simulink model "typeA_export"  (R2017b)
settings: Solver=VariableStepAuto  StartTime=0.0  StopTime=10.0  RelTol=1e-3
values from neighbouring files (symbols this model uses):
  sys1 = sys1_exp    [check_exportvsmake.m]    (also in sumcon2mdlconst_typeA.m = sus.ss)
settings Model: Creator=ayaka  LastModifiedBy=ayaka

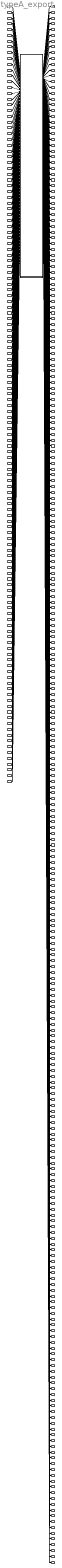
== system typeA_export ==
  axg : Inport
  ayg : Inport  Port=2
  azg : Inport  Port=3
  apitchg : Inport  Port=4
  ayawg : Inport  Port=5
  arollg : Inport  Port=6
  axHLgnd : Inport  Port=7
  ayHLgnd : Inport  Port=8
  azHLgnd : Inport  Port=9
  apitchHLgnd : Inport  Port=10
  ayawHLgnd : Inport  Port=11
  arollHLgnd : Inport  Port=12
  axHLgnd2 : Inport  Port=13
  ayHLgnd2 : Inport  Port=14
  azHLgnd2 : Inport  Port=15
  apitchHLgnd2 : Inport  Port=16
  ayawHLgnd2 : Inport  Port=17
  arollHLgnd2 : Inport  Port=18
  FxF0 : Inport  Port=19
  FzF0 : Inport  Port=20
  FyawF0 : Inport  Port=21
  FxMD : Inport  Port=22
  FyMD : Inport  Port=23
  FzMD : Inport  Port=24
  FpitchMD : Inport  Port=25
  FyawMD : Inport  Port=26
  FrollMD : Inport  Port=27
  FxF1 : Inport  Port=28
  FyF1 : Inport  Port=29
  FzF1 : Inport  Port=30
  FpitchF1 : Inport  Port=31
  FyawF1 : Inport  Port=32
  FrollF1 : Inport  Port=33
  FxF2 : Inport  Port=34
  FyF2 : Inport  Port=35
  FzF2 : Inport  Port=36
  FpitchF2 : Inport  Port=37
  FyawF2 : Inport  Port=38
  FrollF2 : Inport  Port=39
  FxF3 : Inport  Port=40
  FyF3 : Inport  Port=41
  FzF3 : Inport  Port=42
  FpitchF3 : Inport  Port=43
  FyawF3 : Inport  Port=44
  FrollF3 : Inport  Port=45
  FxBF : Inport  Port=46
  FyBF : Inport  Port=47
  FzBF : Inport  Port=48
  FpitchBF : Inport  Port=49
  FyawBF : Inport  Port=50
  FrollBF : Inport  Port=51
  FxPF : Inport  Port=52
  FyPF : Inport  Port=53
  FzPF : Inport  Port=54
  FpitchPF : Inport  Port=55
  FyawPF : Inport  Port=56
  FrollPF : Inport  Port=57
  FxMNR : Inport  Port=58
  FyMNR : Inport  Port=59
  FzMNR : Inport  Port=60
  FpitchMNR : Inport  Port=61
  FyawMNR : Inport  Port=62
  FrollMNR : Inport  Port=63
  FxMN : Inport  Port=64
  FyMN : Inport  Port=65
  FzMN : Inport  Port=66
  FpitchMN : Inport  Port=67
  FyawMN : Inport  Port=68
  FrollMN : Inport  Port=69
  FxIRM : Inport  Port=70
  FyIRM : Inport  Port=71
  FzIRM : Inport  Port=72
  FpitchIRM : Inport  Port=73
  FyawIRM : Inport  Port=74
  FrollIRM : Inport  Port=75
  FxIM : Inport  Port=76
  FyIM : Inport  Port=77
  FzIM : Inport  Port=78
  FpitchIM : Inport  Port=79
  FyawIM : Inport  Port=80
  FrollIM : Inport  Port=81
  FxRM : Inport  Port=82
  FyRM : Inport  Port=83
  FzRM : Inport  Port=84
  FpitchRM : Inport  Port=85
  FyawRM : Inport  Port=86
  FrollRM : Inport  Port=87
  FxTM : Inport  Port=88
  FyTM : Inport  Port=89
  FzTM : Inport  Port=90
  FpitchTM : Inport  Port=91
  FyawTM : Inport  Port=92
  FrollTM : Inport  Port=93
  FxHL1 : Inport  Port=94
  FyHL1 : Inport  Port=95
  FzHL1 : Inport  Port=96
  FpitchHL1 : Inport  Port=97
  FyawHL1 : Inport  Port=98
  FrollHL1 : Inport  Port=99
  FxHL2 : Inport  Port=100
  FyHL2 : Inport  Port=101
  FzHL2 : Inport  Port=102
  FpitchHL2 : Inport  Port=103
  FyawHL2 : Inport  Port=104
  FrollHL2 : Inport  Port=105
  FxHL3 : Inport  Port=106
  FyHL3 : Inport  Port=107
  FzHL3 : Inport  Port=108
  FpitchHL3 : Inport  Port=109
  FyawHL3 : Inport  Port=110
  FrollHL3 : Inport  Port=111
  FxHL21 : Inport  Port=112
  FyHL21 : Inport  Port=113
  FzHL21 : Inport  Port=114
  FpitchHL21 : Inport  Port=115
  FyawHL21 : Inport  Port=116
  FrollHL21 : Inport  Port=117
  FxHL22 : Inport  Port=118
  FyHL22 : Inport  Port=119
  FzHL22 : Inport  Port=120
  FpitchHL22 : Inport  Port=121
  FyawHL22 : Inport  Port=122
  FrollHL22 : Inport  Port=123
  FxHL23 : Inport  Port=124
  FyHL23 : Inport  Port=125
  FzHL23 : Inport  Port=126
  FpitchHL23 : Inport  Port=127
  FyawHL23 : Inport  Port=128
  FrollHL23 : Inport  Port=129
  FxJB : Inport  Port=130
  FyJB : Inport  Port=131
  FzJB : Inport  Port=132
  FpitchJB : Inport  Port=133
  FyawJB : Inport  Port=134
  FrollJB : Inport  Port=135
  Suspension : Subsystem
  xg : Outport
  yg : Outport  Port=2
  zg : Outport  Port=3
  pitchg : Outport  Port=4
  yawg : Outport  Port=5
  rollg : Outport  Port=6
  xHLgnd : Outport  Port=7
  yHLgnd : Outport  Port=8
  zHLgnd : Outport  Port=9
  pitchHLgnd : Outport  Port=10
  yawHLgnd : Outport  Port=11
  rollHLgnd : Outport  Port=12
  xHLgnd2 : Outport  Port=13
  yHLgnd2 : Outport  Port=14
  zHLgnd2 : Outport  Port=15
  pitchHLgnd2 : Outport  Port=16
  yawHLgnd2 : Outport  Port=17
  rollHLgnd2 : Outport  Port=18
  vxg : Outport  Port=19
  vyg : Outport  Port=20
  vzg : Outport  Port=21
  vpitchg : Outport  Port=22
  vyawg : Outport  Port=23
  vrollg : Outport  Port=24
  vxHLgnd : Outport  Port=25
  vyHLgnd : Outport  Port=26
  vzHLgnd : Outport  Port=27
  vpitchHLgnd : Outport  Port=28
  vyawHLgnd : Outport  Port=29
  vrollHLgnd : Outport  Port=30
  vxHLgnd2 : Outport  Port=31
  vyHLgnd2 : Outport  Port=32
  vzHLgnd2 : Outport  Port=33
  vpitchHLgnd2 : Outport  Port=34
  vyawHLgnd2 : Outport  Port=35
  vrollHLgnd2 : Outport  Port=36
  xF0 : Outport  Port=37
  zF0 : Outport  Port=38
  yawF0 : Outport  Port=39
  xMD : Outport  Port=40
  yMD : Outport  Port=41
  zMD : Outport  Port=42
  pitchMD : Outport  Port=43
  yawMD : Outport  Port=44
  rollMD : Outport  Port=45
  xF1 : Outport  Port=46
  yF1 : Outport  Port=47
  zF1 : Outport  Port=48
  pitchF1 : Outport  Port=49
  yawF1 : Outport  Port=50
  rollF1 : Outport  Port=51
  xF2 : Outport  Port=52
  yF2 : Outport  Port=53
  zF2 : Outport  Port=54
  pitchF2 : Outport  Port=55
  yawF2 : Outport  Port=56
  rollF2 : Outport  Port=57
  xF3 : Outport  Port=58
  yF3 : Outport  Port=59
  zF3 : Outport  Port=60
  pitchF3 : Outport  Port=61
  yawF3 : Outport  Port=62
  rollF3 : Outport  Port=63
  xBF : Outport  Port=64
  yBF : Outport  Port=65
  zBF : Outport  Port=66
  pitchBF : Outport  Port=67
  yawBF : Outport  Port=68
  rollBF : Outport  Port=69
  xPF : Outport  Port=70
  yPF : Outport  Port=71
  zPF : Outport  Port=72
  pitchPF : Outport  Port=73
  yawPF : Outport  Port=74
  rollPF : Outport  Port=75
  xMNR : Outport  Port=76
  yMNR : Outport  Port=77
  zMNR : Outport  Port=78
  pitchMNR : Outport  Port=79
  yawMNR : Outport  Port=80
  rollMNR : Outport  Port=81
  xMN : Outport  Port=82
  yMN : Outport  Port=83
  zMN : Outport  Port=84
  pitchMN : Outport  Port=85
  yawMN : Outport  Port=86
  rollMN : Outport  Port=87
  xIRM : Outport  Port=88
  yIRM : Outport  Port=89
  zIRM : Outport  Port=90
  pitchIRM : Outport  Port=91
  yawIRM : Outport  Port=92
  rollIRM : Outport  Port=93
  xIM : Outport  Port=94
  yIM : Outport  Port=95
  zIM : Outport  Port=96
  pitchIM : Outport  Port=97
  yawIM : Outport  Port=98
  rollIM : Outport  Port=99
  xRM : Outport  Port=100
  yRM : Outport  Port=101
  zRM : Outport  Port=102
  pitchRM : Outport  Port=103
  yawRM : Outport  Port=104
  rollRM : Outport  Port=105
  xTM : Outport  Port=106
  yTM : Outport  Port=107
  zTM : Outport  Port=108
  pitchTM : Outport  Port=109
  yawTM : Outport  Port=110
  rollTM : Outport  Port=111
  xHL1 : Outport  Port=112
  yHL1 : Outport  Port=113
  zHL1 : Outport  Port=114
  pitchHL1 : Outport  Port=115
  yawHL1 : Outport  Port=116
  rollHL1 : Outport  Port=117
  xHL2 : Outport  Port=118
  yHL2 : Outport  Port=119
  zHL2 : Outport  Port=120
  pitchHL2 : Outport  Port=121
  yawHL2 : Outport  Port=122
  rollHL2 : Outport  Port=123
  xHL3 : Outport  Port=124
  yHL3 : Outport  Port=125
  zHL3 : Outport  Port=126
  pitchHL3 : Outport  Port=127
  yawHL3 : Outport  Port=128
  rollHL3 : Outport  Port=129
  xHL21 : Outport  Port=130
  yHL21 : Outport  Port=131
  zHL21 : Outport  Port=132
  pitchHL21 : Outport  Port=133
  yawHL21 : Outport  Port=134
  rollHL21 : Outport  Port=135
  xHL22 : Outport  Port=136
  yHL22 : Outport  Port=137
  zHL22 : Outport  Port=138
  pitchHL22 : Outport  Port=139
  yawHL22 : Outport  Port=140
  rollHL22 : Outport  Port=141
  xHL23 : Outport  Port=142
  yHL23 : Outport  Port=143
  zHL23 : Outport  Port=144
  pitchHL23 : Outport  Port=145
  yawHL23 : Outport  Port=146
  rollHL23 : Outport  Port=147
  xJB : Outport  Port=148
  yJB : Outport  Port=149
  zJB : Outport  Port=150
  pitchJB : Outport  Port=151
  yawJB : Outport  Port=152
  rollJB : Outport  Port=153
  vxF0 : Outport  Port=154
  vzF0 : Outport  Port=155
  vyawF0 : Outport  Port=156
  vxMD : Outport  Port=157
  vyMD : Outport  Port=158
  vzMD : Outport  Port=159
  vpitchMD : Outport  Port=160
  vyawMD : Outport  Port=161
  vrollMD : Outport  Port=162
  vxF1 : Outport  Port=163
  vyF1 : Outport  Port=164
  vzF1 : Outport  Port=165
  vpitchF1 : Outport  Port=166
  vyawF1 : Outport  Port=167
  vrollF1 : Outport  Port=168
  vxF2 : Outport  Port=169
  vyF2 : Outport  Port=170
  vzF2 : Outport  Port=171
  vpitchF2 : Outport  Port=172
  vyawF2 : Outport  Port=173
  vrollF2 : Outport  Port=174
  vxF3 : Outport  Port=175
  vyF3 : Outport  Port=176
  vzF3 : Outport  Port=177
  vpitchF3 : Outport  Port=178
  vyawF3 : Outport  Port=179
  vrollF3 : Outport  Port=180
  vxBF : Outport  Port=181
  vyBF : Outport  Port=182
  vzBF : Outport  Port=183
  vpitchBF : Outport  Port=184
  vyawBF : Outport  Port=185
  vrollBF : Outport  Port=186
  vxPF : Outport  Port=187
  vyPF : Outport  Port=188
  vzPF : Outport  Port=189
  vpitchPF : Outport  Port=190
  vyawPF : Outport  Port=191
  vrollPF : Outport  Port=192
  vxMNR : Outport  Port=193
  vyMNR : Outport  Port=194
  vzMNR : Outport  Port=195
  vpitchMNR : Outport  Port=196
  vyawMNR : Outport  Port=197
  vrollMNR : Outport  Port=198
  vxMN : Outport  Port=199
  vyMN : Outport  Port=200
  vzMN : Outport  Port=201
  vpitchMN : Outport  Port=202
  vyawMN : Outport  Port=203
  vrollMN : Outport  Port=204
  vxIRM : Outport  Port=205
  vyIRM : Outport  Port=206
  vzIRM : Outport  Port=207
  vpitchIRM : Outport  Port=208
  vyawIRM : Outport  Port=209
  vrollIRM : Outport  Port=210
  vxIM : Outport  Port=211
  vyIM : Outport  Port=212
  vzIM : Outport  Port=213
  vpitchIM : Outport  Port=214
  vyawIM : Outport  Port=215
  vrollIM : Outport  Port=216
  vxRM : Outport  Port=217
  vyRM : Outport  Port=218
  vzRM : Outport  Port=219
  vpitchRM : Outport  Port=220
  vyawRM : Outport  Port=221
  vrollRM : Outport  Port=222
  vxTM : Outport  Port=223
  vyTM : Outport  Port=224
  vzTM : Outport  Port=225
  vpitchTM : Outport  Port=226
  vyawTM : Outport  Port=227
  vrollTM : Outport  Port=228
  vxHL1 : Outport  Port=229
  vyHL1 : Outport  Port=230
  vzHL1 : Outport  Port=231
  vpitchHL1 : Outport  Port=232
  vyawHL1 : Outport  Port=233
  vrollHL1 : Outport  Port=234
  vxHL2 : Outport  Port=235
  vyHL2 : Outport  Port=236
  vzHL2 : Outport  Port=237
  vpitchHL2 : Outport  Port=238
  vyawHL2 : Outport  Port=239
  vrollHL2 : Outport  Port=240
  vxHL3 : Outport  Port=241
  vyHL3 : Outport  Port=242
  vzHL3 : Outport  Port=243
  vpitchHL3 : Outport  Port=244
  vyawHL3 : Outport  Port=245
  vrollHL3 : Outport  Port=246
  vxHL21 : Outport  Port=247
  vyHL21 : Outport  Port=248
  vzHL21 : Outport  Port=249
  vpitchHL21 : Outport  Port=250
  vyawHL21 : Outport  Port=251
  vrollHL21 : Outport  Port=252
  vxHL22 : Outport  Port=253
  vyHL22 : Outport  Port=254
  vzHL22 : Outport  Port=255
  vpitchHL22 : Outport  Port=256
  vyawHL22 : Outport  Port=257
  vrollHL22 : Outport  Port=258
  vxHL23 : Outport  Port=259
  vyHL23 : Outport  Port=260
  vzHL23 : Outport  Port=261
  vpitchHL23 : Outport  Port=262
  vyawHL23 : Outport  Port=263
  vrollHL23 : Outport  Port=264
  vxJB : Outport  Port=265
  vyJB : Outport  Port=266
  vzJB : Outport  Port=267
  vpitchJB : Outport  Port=268
  vyawJB : Outport  Port=269
  vrollJB : Outport  Port=270
  wires:
  axg/1 -> Suspension/1(axg)
  ayg/1 -> Suspension/2(ayg)
  azg/1 -> Suspension/3(azg)
  apitchg/1 -> Suspension/4(apitchg)
  ayawg/1 -> Suspension/5(ayawg)
  arollg/1 -> Suspension/6(arollg)
  axHLgnd/1 -> Suspension/7(axHLgnd)
  ayHLgnd/1 -> Suspension/8(ayHLgnd)
  azHLgnd/1 -> Suspension/9(azHLgnd)
  apitchHLgnd/1 -> Suspension/10(apitchHLgnd)
  ayawHLgnd/1 -> Suspension/11(ayawHLgnd)
  arollHLgnd/1 -> Suspension/12(arollHLgnd)
  axHLgnd2/1 -> Suspension/13(axHLgnd2)
  ayHLgnd2/1 -> Suspension/14(ayHLgnd2)
  azHLgnd2/1 -> Suspension/15(azHLgnd2)
  apitchHLgnd2/1 -> Suspension/16(apitchHLgnd2)
  ayawHLgnd2/1 -> Suspension/17(ayawHLgnd2)
  arollHLgnd2/1 -> Suspension/18(arollHLgnd2)
  FxF0/1 -> Suspension/19(FxF0)
  FzF0/1 -> Suspension/20(FzF0)
  FyawF0/1 -> Suspension/21(FyawF0)
  FxMD/1 -> Suspension/22(FxMD)
  FyMD/1 -> Suspension/23(FyMD)
  FzMD/1 -> Suspension/24(FzMD)
  FpitchMD/1 -> Suspension/25(FpitchMD)
  FyawMD/1 -> Suspension/26(FyawMD)
  FrollMD/1 -> Suspension/27(FrollMD)
  FxF1/1 -> Suspension/28(FxF1)
  FyF1/1 -> Suspension/29(FyF1)
  FzF1/1 -> Suspension/30(FzF1)
  FpitchF1/1 -> Suspension/31(FpitchF1)
  FyawF1/1 -> Suspension/32(FyawF1)
  FrollF1/1 -> Suspension/33(FrollF1)
  FxF2/1 -> Suspension/34(FxF2)
  FyF2/1 -> Suspension/35(FyF2)
  FzF2/1 -> Suspension/36(FzF2)
  FpitchF2/1 -> Suspension/37(FpitchF2)
  FyawF2/1 -> Suspension/38(FyawF2)
  FrollF2/1 -> Suspension/39(FrollF2)
  FxF3/1 -> Suspension/40(FxF3)
  FyF3/1 -> Suspension/41(FyF3)
  FzF3/1 -> Suspension/42(FzF3)
  FpitchF3/1 -> Suspension/43(FpitchF3)
  FyawF3/1 -> Suspension/44(FyawF3)
  FrollF3/1 -> Suspension/45(FrollF3)
  FxBF/1 -> Suspension/46(FxBF)
  FyBF/1 -> Suspension/47(FyBF)
  FzBF/1 -> Suspension/48(FzBF)
  FpitchBF/1 -> Suspension/49(FpitchBF)
  FyawBF/1 -> Suspension/50(FyawBF)
  FrollBF/1 -> Suspension/51(FrollBF)
  FxPF/1 -> Suspension/52(FxPF)
  FyPF/1 -> Suspension/53(FyPF)
  FzPF/1 -> Suspension/54(FzPF)
  FpitchPF/1 -> Suspension/55(FpitchPF)
  FyawPF/1 -> Suspension/56(FyawPF)
  FrollPF/1 -> Suspension/57(FrollPF)
  FxMNR/1 -> Suspension/58(FxMNR)
  FyMNR/1 -> Suspension/59(FyMNR)
  FzMNR/1 -> Suspension/60(FzMNR)
  FpitchMNR/1 -> Suspension/61(FpitchMNR)
  FyawMNR/1 -> Suspension/62(FyawMNR)
  FrollMNR/1 -> Suspension/63(FrollMNR)
  FxMN/1 -> Suspension/64(FxMN)
  FyMN/1 -> Suspension/65(FyMN)
  FzMN/1 -> Suspension/66(FzMN)
  FpitchMN/1 -> Suspension/67(FpitchMN)
  FyawMN/1 -> Suspension/68(FyawMN)
  FrollMN/1 -> Suspension/69(FrollMN)
  FxIRM/1 -> Suspension/70(FxIRM)
  FyIRM/1 -> Suspension/71(FyIRM)
  FzIRM/1 -> Suspension/72(FzIRM)
  FpitchIRM/1 -> Suspension/73(FpitchIRM)
  FyawIRM/1 -> Suspension/74(FyawIRM)
  FrollIRM/1 -> Suspension/75(FrollIRM)
  FxIM/1 -> Suspension/76(FxIM)
  FyIM/1 -> Suspension/77(FyIM)
  FzIM/1 -> Suspension/78(FzIM)
  FpitchIM/1 -> Suspension/79(FpitchIM)
  FyawIM/1 -> Suspension/80(FyawIM)
  FrollIM/1 -> Suspension/81(FrollIM)
  FxRM/1 -> Suspension/82(FxRM)
  FyRM/1 -> Suspension/83(FyRM)
  FzRM/1 -> Suspension/84(FzRM)
  FpitchRM/1 -> Suspension/85(FpitchRM)
  FyawRM/1 -> Suspension/86(FyawRM)
  FrollRM/1 -> Suspension/87(FrollRM)
  FxTM/1 -> Suspension/88(FxTM)
  FyTM/1 -> Suspension/89(FyTM)
  FzTM/1 -> Suspension/90(FzTM)
  FpitchTM/1 -> Suspension/91(FpitchTM)
  FyawTM/1 -> Suspension/92(FyawTM)
  FrollTM/1 -> Suspension/93(FrollTM)
  FxHL1/1 -> Suspension/94(FxHL1)
  FyHL1/1 -> Suspension/95(FyHL1)
  FzHL1/1 -> Suspension/96(FzHL1)
  FpitchHL1/1 -> Suspension/97(FpitchHL1)
  FyawHL1/1 -> Suspension/98(FyawHL1)
  FrollHL1/1 -> Suspension/99(FrollHL1)
  FxHL2/1 -> Suspension/100(FxHL2)
  FyHL2/1 -> Suspension/101(FyHL2)
  FzHL2/1 -> Suspension/102(FzHL2)
  FpitchHL2/1 -> Suspension/103(FpitchHL2)
  FyawHL2/1 -> Suspension/104(FyawHL2)
  FrollHL2/1 -> Suspension/105(FrollHL2)
  FxHL3/1 -> Suspension/106(FxHL3)
  FyHL3/1 -> Suspension/107(FyHL3)
  FzHL3/1 -> Suspension/108(FzHL3)
  FpitchHL3/1 -> Suspension/109(FpitchHL3)
  FyawHL3/1 -> Suspension/110(FyawHL3)
  FrollHL3/1 -> Suspension/111(FrollHL3)
  FxHL21/1 -> Suspension/112(FxHL21)
  FyHL21/1 -> Suspension/113(FyHL21)
  FzHL21/1 -> Suspension/114(FzHL21)
  FpitchHL21/1 -> Suspension/115(FpitchHL21)
  FyawHL21/1 -> Suspension/116(FyawHL21)
  FrollHL21/1 -> Suspension/117(FrollHL21)
  FxHL22/1 -> Suspension/118(FxHL22)
  FyHL22/1 -> Suspension/119(FyHL22)
  FzHL22/1 -> Suspension/120(FzHL22)
  FpitchHL22/1 -> Suspension/121(FpitchHL22)
  FyawHL22/1 -> Suspension/122(FyawHL22)
  FrollHL22/1 -> Suspension/123(FrollHL22)
  FxHL23/1 -> Suspension/124(FxHL23)
  FyHL23/1 -> Suspension/125(FyHL23)
  FzHL23/1 -> Suspension/126(FzHL23)
  FpitchHL23/1 -> Suspension/127(FpitchHL23)
  FyawHL23/1 -> Suspension/128(FyawHL23)
  FrollHL23/1 -> Suspension/129(FrollHL23)
  FxJB/1 -> Suspension/130(FxJB)
  FyJB/1 -> Suspension/131(FyJB)
  FzJB/1 -> Suspension/132(FzJB)
  FpitchJB/1 -> Suspension/133(FpitchJB)
  FyawJB/1 -> Suspension/134(FyawJB)
  FrollJB/1 -> Suspension/135(FrollJB)
  Suspension/1(xg) -> xg/1
  Suspension/2(yg) -> yg/1
  Suspension/3(zg) -> zg/1
  Suspension/4(pitchg) -> pitchg/1
  Suspension/5(yawg) -> yawg/1
  Suspension/6(rollg) -> rollg/1
  Suspension/7(xHLgnd) -> xHLgnd/1
  Suspension/8(yHLgnd) -> yHLgnd/1
  Suspension/9(zHLgnd) -> zHLgnd/1
  Suspension/10(pitchHLgnd) -> pitchHLgnd/1
  Suspension/11(yawHLgnd) -> yawHLgnd/1
  Suspension/12(rollHLgnd) -> rollHLgnd/1
  Suspension/13(xHLgnd2) -> xHLgnd2/1
  Suspension/14(yHLgnd2) -> yHLgnd2/1
  Suspension/15(zHLgnd2) -> zHLgnd2/1
  Suspension/16(pitchHLgnd2) -> pitchHLgnd2/1
  Suspension/17(yawHLgnd2) -> yawHLgnd2/1
  Suspension/18(rollHLgnd2) -> rollHLgnd2/1
  Suspension/19(vxg) -> vxg/1
  Suspension/20(vyg) -> vyg/1
  Suspension/21(vzg) -> vzg/1
  Suspension/22(vpitchg) -> vpitchg/1
  Suspension/23(vyawg) -> vyawg/1
  Suspension/24(vrollg) -> vrollg/1
  Suspension/25(vxHLgnd) -> vxHLgnd/1
  Suspension/26(vyHLgnd) -> vyHLgnd/1
  Suspension/27(vzHLgnd) -> vzHLgnd/1
  Suspension/28(vpitchHLgnd) -> vpitchHLgnd/1
  Suspension/29(vyawHLgnd) -> vyawHLgnd/1
  Suspension/30(vrollHLgnd) -> vrollHLgnd/1
  Suspension/31(vxHLgnd2) -> vxHLgnd2/1
  Suspension/32(vyHLgnd2) -> vyHLgnd2/1
  Suspension/33(vzHLgnd2) -> vzHLgnd2/1
  Suspension/34(vpitchHLgnd2) -> vpitchHLgnd2/1
  Suspension/35(vyawHLgnd2) -> vyawHLgnd2/1
  Suspension/36(vrollHLgnd2) -> vrollHLgnd2/1
  Suspension/37(xF0) -> xF0/1
  Suspension/38(zF0) -> zF0/1
  Suspension/39(yawF0) -> yawF0/1
  Suspension/40(xMD) -> xMD/1
  Suspension/41(yMD) -> yMD/1
  Suspension/42(zMD) -> zMD/1
  Suspension/43(pitchMD) -> pitchMD/1
  Suspension/44(yawMD) -> yawMD/1
  Suspension/45(rollMD) -> rollMD/1
  Suspension/46(xF1) -> xF1/1
  Suspension/47(yF1) -> yF1/1
  Suspension/48(zF1) -> zF1/1
  Suspension/49(pitchF1) -> pitchF1/1
  Suspension/50(yawF1) -> yawF1/1
  Suspension/51(rollF1) -> rollF1/1
  Suspension/52(xF2) -> xF2/1
  Suspension/53(yF2) -> yF2/1
  Suspension/54(zF2) -> zF2/1
  Suspension/55(pitchF2) -> pitchF2/1
  Suspension/56(yawF2) -> yawF2/1
  Suspension/57(rollF2) -> rollF2/1
  Suspension/58(xF3) -> xF3/1
  Suspension/59(yF3) -> yF3/1
  Suspension/60(zF3) -> zF3/1
  Suspension/61(pitchF3) -> pitchF3/1
  Suspension/62(yawF3) -> yawF3/1
  Suspension/63(rollF3) -> rollF3/1
  Suspension/64(xBF) -> xBF/1
  Suspension/65(yBF) -> yBF/1
  Suspension/66(zBF) -> zBF/1
  Suspension/67(pitchBF) -> pitchBF/1
  Suspension/68(yawBF) -> yawBF/1
  Suspension/69(rollBF) -> rollBF/1
  Suspension/70(xPF) -> xPF/1
  Suspension/71(yPF) -> yPF/1
  Suspension/72(zPF) -> zPF/1
  Suspension/73(pitchPF) -> pitchPF/1
  Suspension/74(yawPF) -> yawPF/1
  Suspension/75(rollPF) -> rollPF/1
  Suspension/76(xMNR) -> xMNR/1
  Suspension/77(yMNR) -> yMNR/1
  Suspension/78(zMNR) -> zMNR/1
  Suspension/79(pitchMNR) -> pitchMNR/1
  Suspension/80(yawMNR) -> yawMNR/1
  Suspension/81(rollMNR) -> rollMNR/1
  Suspension/82(xMN) -> xMN/1
  Suspension/83(yMN) -> yMN/1
  Suspension/84(zMN) -> zMN/1
  Suspension/85(pitchMN) -> pitchMN/1
  Suspension/86(yawMN) -> yawMN/1
  Suspension/87(rollMN) -> rollMN/1
  Suspension/88(xIRM) -> xIRM/1
  Suspension/89(yIRM) -> yIRM/1
  Suspension/90(zIRM) -> zIRM/1
  Suspension/91(pitchIRM) -> pitchIRM/1
  Suspension/92(yawIRM) -> yawIRM/1
  Suspension/93(rollIRM) -> rollIRM/1
  Suspension/94(xIM) -> xIM/1
  Suspension/95(yIM) -> yIM/1
  Suspension/96(zIM) -> zIM/1
  Suspension/97(pitchIM) -> pitchIM/1
  Suspension/98(yawIM) -> yawIM/1
  Suspension/99(rollIM) -> rollIM/1
  Suspension/100(xRM) -> xRM/1
  Suspension/101(yRM) -> yRM/1
  Suspension/102(zRM) -> zRM/1
  Suspension/103(pitchRM) -> pitchRM/1
  Suspension/104(yawRM) -> yawRM/1
  Suspension/105(rollRM) -> rollRM/1
  Suspension/106(xTM) -> xTM/1
  Suspension/107(yTM) -> yTM/1
  Suspension/108(zTM) -> zTM/1
  Suspension/109(pitchTM) -> pitchTM/1
  Suspension/110(yawTM) -> yawTM/1
  Suspension/111(rollTM) -> rollTM/1
  Suspension/112(xHL1) -> xHL1/1
  Suspension/113(yHL1) -> yHL1/1
  Suspension/114(zHL1) -> zHL1/1
  Suspension/115(pitchHL1) -> pitchHL1/1
  Suspension/116(yawHL1) -> yawHL1/1
  Suspension/117(rollHL1) -> rollHL1/1
  Suspension/118(xHL2) -> xHL2/1
  Suspension/119(yHL2) -> yHL2/1
  Suspension/120(zHL2) -> zHL2/1
  Suspension/121(pitchHL2) -> pitchHL2/1
  Suspension/122(yawHL2) -> yawHL2/1
  Suspension/123(rollHL2) -> rollHL2/1
  Suspension/124(xHL3) -> xHL3/1
  Suspension/125(yHL3) -> yHL3/1
  Suspension/126(zHL3) -> zHL3/1
  Suspension/127(pitchHL3) -> pitchHL3/1
  Suspension/128(yawHL3) -> yawHL3/1
  Suspension/129(rollHL3) -> rollHL3/1
  Suspension/130(xHL21) -> xHL21/1
  Suspension/131(yHL21) -> yHL21/1
  Suspension/132(zHL21) -> zHL21/1
  Suspension/133(pitchHL21) -> pitchHL21/1
  Suspension/134(yawHL21) -> yawHL21/1
  Suspension/135(rollHL21) -> rollHL21/1
  Suspension/136(xHL22) -> xHL22/1
  Suspension/137(yHL22) -> yHL22/1
  Suspension/138(zHL22) -> zHL22/1
  Suspension/139(pitchHL22) -> pitchHL22/1
  Suspension/140(yawHL22) -> yawHL22/1
  Suspension/141(rollHL22) -> rollHL22/1
  Suspension/142(xHL23) -> xHL23/1
  Suspension/143(yHL23) -> yHL23/1
  Suspension/144(zHL23) -> zHL23/1
  Suspension/145(pitchHL23) -> pitchHL23/1
  Suspension/146(yawHL23) -> yawHL23/1
  Suspension/147(rollHL23) -> rollHL23/1
  Suspension/148(xJB) -> xJB/1
  Suspension/149(yJB) -> yJB/1
  Suspension/150(zJB) -> zJB/1
  Suspension/151(pitchJB) -> pitchJB/1
  Suspension/152(yawJB) -> yawJB/1
  Suspension/153(rollJB) -> rollJB/1
  Suspension/154(vxF0) -> vxF0/1
  Suspension/155(vzF0) -> vzF0/1
  Suspension/156(vyawF0) -> vyawF0/1
  Suspension/157(vxMD) -> vxMD/1
  Suspension/158(vyMD) -> vyMD/1
  Suspension/159(vzMD) -> vzMD/1
  Suspension/160(vpitchMD) -> vpitchMD/1
  Suspension/161(vyawMD) -> vyawMD/1
  Suspension/162(vrollMD) -> vrollMD/1
  Suspension/163(vxF1) -> vxF1/1
  Suspension/164(vyF1) -> vyF1/1
  Suspension/165(vzF1) -> vzF1/1
  Suspension/166(vpitchF1) -> vpitchF1/1
  Suspension/167(vyawF1) -> vyawF1/1
  Suspension/168(vrollF1) -> vrollF1/1
  Suspension/169(vxF2) -> vxF2/1
  Suspension/170(vyF2) -> vyF2/1
  Suspension/171(vzF2) -> vzF2/1
  Suspension/172(vpitchF2) -> vpitchF2/1
  Suspension/173(vyawF2) -> vyawF2/1
  Suspension/174(vrollF2) -> vrollF2/1
  Suspension/175(vxF3) -> vxF3/1
  Suspension/176(vyF3) -> vyF3/1
  Suspension/177(vzF3) -> vzF3/1
  Suspension/178(vpitchF3) -> vpitchF3/1
  Suspension/179(vyawF3) -> vyawF3/1
  Suspension/180(vrollF3) -> vrollF3/1
  Suspension/181(vxBF) -> vxBF/1
  Suspension/182(vyBF) -> vyBF/1
  Suspension/183(vzBF) -> vzBF/1
  Suspension/184(vpitchBF) -> vpitchBF/1
  Suspension/185(vyawBF) -> vyawBF/1
  Suspension/186(vrollBF) -> vrollBF/1
  Suspension/187(vxPF) -> vxPF/1
  Suspension/188(vyPF) -> vyPF/1
  Suspension/189(vzPF) -> vzPF/1
  Suspension/190(vpitchPF) -> vpitchPF/1
  Suspension/191(vyawPF) -> vyawPF/1
  Suspension/192(vrollPF) -> vrollPF/1
  Suspension/193(vxMNR) -> vxMNR/1
  Suspension/194(vyMNR) -> vyMNR/1
  Suspension/195(vzMNR) -> vzMNR/1
  Suspension/196(vpitchMNR) -> vpitchMNR/1
  Suspension/197(vyawMNR) -> vyawMNR/1
  Suspension/198(vrollMNR) -> vrollMNR/1
  Suspension/199(vxMN) -> vxMN/1
  Suspension/200(vyMN) -> vyMN/1
  Suspension/201(vzMN) -> vzMN/1
  Suspension/202(vpitchMN) -> vpitchMN/1
  Suspension/203(vyawMN) -> vyawMN/1
  Suspension/204(vrollMN) -> vrollMN/1
  Suspension/205(vxIRM) -> vxIRM/1
  Suspension/206(vyIRM) -> vyIRM/1
  Suspension/207(vzIRM) -> vzIRM/1
  Suspension/208(vpitchIRM) -> vpitchIRM/1
  Suspension/209(vyawIRM) -> vyawIRM/1
  Suspension/210(vrollIRM) -> vrollIRM/1
  Suspension/211(vxIM) -> vxIM/1
  Suspension/212(vyIM) -> vyIM/1
  Suspension/213(vzIM) -> vzIM/1
  Suspension/214(vpitchIM) -> vpitchIM/1
  Suspension/215(vyawIM) -> vyawIM/1
  Suspension/216(vrollIM) -> vrollIM/1
  Suspension/217(vxRM) -> vxRM/1
  Suspension/218(vyRM) -> vyRM/1
  Suspension/219(vzRM) -> vzRM/1
  Suspension/220(vpitchRM) -> vpitchRM/1
  Suspension/221(vyawRM) -> vyawRM/1
  Suspension/222(vrollRM) -> vrollRM/1
  Suspension/223(vxTM) -> vxTM/1
  Suspension/224(vyTM) -> vyTM/1
  Suspension/225(vzTM) -> vzTM/1
  Suspension/226(vpitchTM) -> vpitchTM/1
  Suspension/227(vyawTM) -> vyawTM/1
  Suspension/228(vrollTM) -> vrollTM/1
  Suspension/229(vxHL1) -> vxHL1/1
  Suspension/230(vyHL1) -> vyHL1/1
  Suspension/231(vzHL1) -> vzHL1/1
  Suspension/232(vpitchHL1) -> vpitchHL1/1
  Suspension/233(vyawHL1) -> vyawHL1/1
  Suspension/234(vrollHL1) -> vrollHL1/1
  Suspension/235(vxHL2) -> vxHL2/1
  Suspension/236(vyHL2) -> vyHL2/1
  Suspension/237(vzHL2) -> vzHL2/1
  Suspension/238(vpitchHL2) -> vpitchHL2/1
  Suspension/239(vyawHL2) -> vyawHL2/1
  Suspension/240(vrollHL2) -> vrollHL2/1
  Suspension/241(vxHL3) -> vxHL3/1
  Suspension/242(vyHL3) -> vyHL3/1
  Suspension/243(vzHL3) -> vzHL3/1
  Suspension/244(vpitchHL3) -> vpitchHL3/1
  Suspension/245(vyawHL3) -> vyawHL3/1
  Suspension/246(vrollHL3) -> vrollHL3/1
  Suspension/247(vxHL21) -> vxHL21/1
  Suspension/248(vyHL21) -> vyHL21/1
  Suspension/249(vzHL21) -> vzHL21/1
  Suspension/250(vpitchHL21) -> vpitchHL21/1
  Suspension/251(vyawHL21) -> vyawHL21/1
  Suspension/252(vrollHL21) -> vrollHL21/1
  Suspension/253(vxHL22) -> vxHL22/1
  Suspension/254(vyHL22) -> vyHL22/1
  Suspension/255(vzHL22) -> vzHL22/1
  Suspension/256(vpitchHL22) -> vpitchHL22/1
  Suspension/257(vyawHL22) -> vyawHL22/1
  Suspension/258(vrollHL22) -> vrollHL22/1
  Suspension/259(vxHL23) -> vxHL23/1
  Suspension/260(vyHL23) -> vyHL23/1
  Suspension/261(vzHL23) -> vzHL23/1
  Suspension/262(vpitchHL23) -> vpitchHL23/1
  Suspension/263(vyawHL23) -> vyawHL23/1
  Suspension/264(vrollHL23) -> vrollHL23/1
  Suspension/265(vxJB) -> vxJB/1
  Suspension/266(vyJB) -> vyJB/1
  Suspension/267(vzJB) -> vzJB/1
  Suspension/268(vpitchJB) -> vpitchJB/1
  Suspension/269(vyawJB) -> vyawJB/1
  Suspension/270(vrollJB) -> vrollJB/1

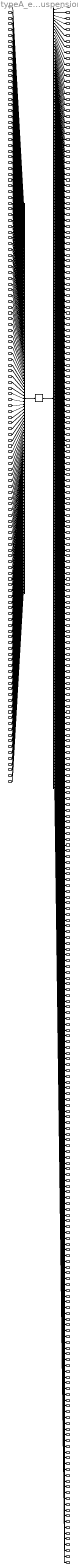
== system typeA_export/Suspension ==
  axg : Inport
  ayg : Inport  Port=2
  azg : Inport  Port=3
  apitchg : Inport  Port=4
  ayawg : Inport  Port=5
  arollg : Inport  Port=6
  axHLgnd : Inport  Port=7
  ayHLgnd : Inport  Port=8
  azHLgnd : Inport  Port=9
  apitchHLgnd : Inport  Port=10
  ayawHLgnd : Inport  Port=11
  arollHLgnd : Inport  Port=12
  axHLgnd2 : Inport  Port=13
  ayHLgnd2 : Inport  Port=14
  azHLgnd2 : Inport  Port=15
  apitchHLgnd2 : Inport  Port=16
  ayawHLgnd2 : Inport  Port=17
  arollHLgnd2 : Inport  Port=18
  FxF0 : Inport  Port=19
  FzF0 : Inport  Port=20
  FyawF0 : Inport  Port=21
  FxMD : Inport  Port=22
  FyMD : Inport  Port=23
  FzMD : Inport  Port=24
  FpitchMD : Inport  Port=25
  FyawMD : Inport  Port=26
  FrollMD : Inport  Port=27
  FxF1 : Inport  Port=28
  FyF1 : Inport  Port=29
  FzF1 : Inport  Port=30
  FpitchF1 : Inport  Port=31
  FyawF1 : Inport  Port=32
  FrollF1 : Inport  Port=33
  FxF2 : Inport  Port=34
  FyF2 : Inport  Port=35
  FzF2 : Inport  Port=36
  FpitchF2 : Inport  Port=37
  FyawF2 : Inport  Port=38
  FrollF2 : Inport  Port=39
  FxF3 : Inport  Port=40
  FyF3 : Inport  Port=41
  FzF3 : Inport  Port=42
  FpitchF3 : Inport  Port=43
  FyawF3 : Inport  Port=44
  FrollF3 : Inport  Port=45
  FxBF : Inport  Port=46
  FyBF : Inport  Port=47
  FzBF : Inport  Port=48
  FpitchBF : Inport  Port=49
  FyawBF : Inport  Port=50
  FrollBF : Inport  Port=51
  FxPF : Inport  Port=52
  FyPF : Inport  Port=53
  FzPF : Inport  Port=54
  FpitchPF : Inport  Port=55
  FyawPF : Inport  Port=56
  FrollPF : Inport  Port=57
  FxMNR : Inport  Port=58
  FyMNR : Inport  Port=59
  FzMNR : Inport  Port=60
  FpitchMNR : Inport  Port=61
  FyawMNR : Inport  Port=62
  FrollMNR : Inport  Port=63
  FxMN : Inport  Port=64
  FyMN : Inport  Port=65
  FzMN : Inport  Port=66
  FpitchMN : Inport  Port=67
  FyawMN : Inport  Port=68
  FrollMN : Inport  Port=69
  FxIRM : Inport  Port=70
  FyIRM : Inport  Port=71
  FzIRM : Inport  Port=72
  FpitchIRM : Inport  Port=73
  FyawIRM : Inport  Port=74
  FrollIRM : Inport  Port=75
  FxIM : Inport  Port=76
  FyIM : Inport  Port=77
  FzIM : Inport  Port=78
  FpitchIM : Inport  Port=79
  FyawIM : Inport  Port=80
  FrollIM : Inport  Port=81
  FxRM : Inport  Port=82
  FyRM : Inport  Port=83
  FzRM : Inport  Port=84
  FpitchRM : Inport  Port=85
  FyawRM : Inport  Port=86
  FrollRM : Inport  Port=87
  FxTM : Inport  Port=88
  FyTM : Inport  Port=89
  FzTM : Inport  Port=90
  FpitchTM : Inport  Port=91
  FyawTM : Inport  Port=92
  FrollTM : Inport  Port=93
  FxHL1 : Inport  Port=94
  FyHL1 : Inport  Port=95
  FzHL1 : Inport  Port=96
  FpitchHL1 : Inport  Port=97
  FyawHL1 : Inport  Port=98
  FrollHL1 : Inport  Port=99
  FxHL2 : Inport  Port=100
  FyHL2 : Inport  Port=101
  FzHL2 : Inport  Port=102
  FpitchHL2 : Inport  Port=103
  FyawHL2 : Inport  Port=104
  FrollHL2 : Inport  Port=105
  FxHL3 : Inport  Port=106
  FyHL3 : Inport  Port=107
  FzHL3 : Inport  Port=108
  FpitchHL3 : Inport  Port=109
  FyawHL3 : Inport  Port=110
  FrollHL3 : Inport  Port=111
  FxHL21 : Inport  Port=112
  FyHL21 : Inport  Port=113
  FzHL21 : Inport  Port=114
  FpitchHL21 : Inport  Port=115
  FyawHL21 : Inport  Port=116
  FrollHL21 : Inport  Port=117
  FxHL22 : Inport  Port=118
  FyHL22 : Inport  Port=119
  FzHL22 : Inport  Port=120
  FpitchHL22 : Inport  Port=121
  FyawHL22 : Inport  Port=122
  FrollHL22 : Inport  Port=123
  FxHL23 : Inport  Port=124
  FyHL23 : Inport  Port=125
  FzHL23 : Inport  Port=126
  FpitchHL23 : Inport  Port=127
  FyawHL23 : Inport  Port=128
  FrollHL23 : Inport  Port=129
  FxJB : Inport  Port=130
  FyJB : Inport  Port=131
  FzJB : Inport  Port=132
  FpitchJB : Inport  Port=133
  FyawJB : Inport  Port=134
  FrollJB : Inport  Port=135
  SAS State-Space : StateSpace  A=sys1.A  B=sys1.B  C=sys1.C  D=sys1.D  InitialCondition=0  ContinuousStateAttributes='SUS_SS_MODEL'
  demux : Demux  Outputs=270
  mux : Mux  Inputs=135
  xg : Outport
  yg : Outport  Port=2
  zg : Outport  Port=3
  pitchg : Outport  Port=4
  yawg : Outport  Port=5
  rollg : Outport  Port=6
  xHLgnd : Outport  Port=7
  yHLgnd : Outport  Port=8
  zHLgnd : Outport  Port=9
  pitchHLgnd : Outport  Port=10
  yawHLgnd : Outport  Port=11
  rollHLgnd : Outport  Port=12
  xHLgnd2 : Outport  Port=13
  yHLgnd2 : Outport  Port=14
  zHLgnd2 : Outport  Port=15
  pitchHLgnd2 : Outport  Port=16
  yawHLgnd2 : Outport  Port=17
  rollHLgnd2 : Outport  Port=18
  vxg : Outport  Port=19
  vyg : Outport  Port=20
  vzg : Outport  Port=21
  vpitchg : Outport  Port=22
  vyawg : Outport  Port=23
  vrollg : Outport  Port=24
  vxHLgnd : Outport  Port=25
  vyHLgnd : Outport  Port=26
  vzHLgnd : Outport  Port=27
  vpitchHLgnd : Outport  Port=28
  vyawHLgnd : Outport  Port=29
  vrollHLgnd : Outport  Port=30
  vxHLgnd2 : Outport  Port=31
  vyHLgnd2 : Outport  Port=32
  vzHLgnd2 : Outport  Port=33
  vpitchHLgnd2 : Outport  Port=34
  vyawHLgnd2 : Outport  Port=35
  vrollHLgnd2 : Outport  Port=36
  xF0 : Outport  Port=37
  zF0 : Outport  Port=38
  yawF0 : Outport  Port=39
  xMD : Outport  Port=40
  yMD : Outport  Port=41
  zMD : Outport  Port=42
  pitchMD : Outport  Port=43
  yawMD : Outport  Port=44
  rollMD : Outport  Port=45
  xF1 : Outport  Port=46
  yF1 : Outport  Port=47
  zF1 : Outport  Port=48
  pitchF1 : Outport  Port=49
  yawF1 : Outport  Port=50
  rollF1 : Outport  Port=51
  xF2 : Outport  Port=52
  yF2 : Outport  Port=53
  zF2 : Outport  Port=54
  pitchF2 : Outport  Port=55
  yawF2 : Outport  Port=56
  rollF2 : Outport  Port=57
  xF3 : Outport  Port=58
  yF3 : Outport  Port=59
  zF3 : Outport  Port=60
  pitchF3 : Outport  Port=61
  yawF3 : Outport  Port=62
  rollF3 : Outport  Port=63
  xBF : Outport  Port=64
  yBF : Outport  Port=65
  zBF : Outport  Port=66
  pitchBF : Outport  Port=67
  yawBF : Outport  Port=68
  rollBF : Outport  Port=69
  xPF : Outport  Port=70
  yPF : Outport  Port=71
  zPF : Outport  Port=72
  pitchPF : Outport  Port=73
  yawPF : Outport  Port=74
  rollPF : Outport  Port=75
  xMNR : Outport  Port=76
  yMNR : Outport  Port=77
  zMNR : Outport  Port=78
  pitchMNR : Outport  Port=79
  yawMNR : Outport  Port=80
  rollMNR : Outport  Port=81
  xMN : Outport  Port=82
  yMN : Outport  Port=83
  zMN : Outport  Port=84
  pitchMN : Outport  Port=85
  yawMN : Outport  Port=86
  rollMN : Outport  Port=87
  xIRM : Outport  Port=88
  yIRM : Outport  Port=89
  zIRM : Outport  Port=90
  pitchIRM : Outport  Port=91
  yawIRM : Outport  Port=92
  rollIRM : Outport  Port=93
  xIM : Outport  Port=94
  yIM : Outport  Port=95
  zIM : Outport  Port=96
  pitchIM : Outport  Port=97
  yawIM : Outport  Port=98
  rollIM : Outport  Port=99
  xRM : Outport  Port=100
  yRM : Outport  Port=101
  zRM : Outport  Port=102
  pitchRM : Outport  Port=103
  yawRM : Outport  Port=104
  rollRM : Outport  Port=105
  xTM : Outport  Port=106
  yTM : Outport  Port=107
  zTM : Outport  Port=108
  pitchTM : Outport  Port=109
  yawTM : Outport  Port=110
  rollTM : Outport  Port=111
  xHL1 : Outport  Port=112
  yHL1 : Outport  Port=113
  zHL1 : Outport  Port=114
  pitchHL1 : Outport  Port=115
  yawHL1 : Outport  Port=116
  rollHL1 : Outport  Port=117
  xHL2 : Outport  Port=118
  yHL2 : Outport  Port=119
  zHL2 : Outport  Port=120
  pitchHL2 : Outport  Port=121
  yawHL2 : Outport  Port=122
  rollHL2 : Outport  Port=123
  xHL3 : Outport  Port=124
  yHL3 : Outport  Port=125
  zHL3 : Outport  Port=126
  pitchHL3 : Outport  Port=127
  yawHL3 : Outport  Port=128
  rollHL3 : Outport  Port=129
  xHL21 : Outport  Port=130
  yHL21 : Outport  Port=131
  zHL21 : Outport  Port=132
  pitchHL21 : Outport  Port=133
  yawHL21 : Outport  Port=134
  rollHL21 : Outport  Port=135
  xHL22 : Outport  Port=136
  yHL22 : Outport  Port=137
  zHL22 : Outport  Port=138
  pitchHL22 : Outport  Port=139
  yawHL22 : Outport  Port=140
  rollHL22 : Outport  Port=141
  xHL23 : Outport  Port=142
  yHL23 : Outport  Port=143
  zHL23 : Outport  Port=144
  pitchHL23 : Outport  Port=145
  yawHL23 : Outport  Port=146
  rollHL23 : Outport  Port=147
  xJB : Outport  Port=148
  yJB : Outport  Port=149
  zJB : Outport  Port=150
  pitchJB : Outport  Port=151
  yawJB : Outport  Port=152
  rollJB : Outport  Port=153
  vxF0 : Outport  Port=154
  vzF0 : Outport  Port=155
  vyawF0 : Outport  Port=156
  vxMD : Outport  Port=157
  vyMD : Outport  Port=158
  vzMD : Outport  Port=159
  vpitchMD : Outport  Port=160
  vyawMD : Outport  Port=161
  vrollMD : Outport  Port=162
  vxF1 : Outport  Port=163
  vyF1 : Outport  Port=164
  vzF1 : Outport  Port=165
  vpitchF1 : Outport  Port=166
  vyawF1 : Outport  Port=167
  vrollF1 : Outport  Port=168
  vxF2 : Outport  Port=169
  vyF2 : Outport  Port=170
  vzF2 : Outport  Port=171
  vpitchF2 : Outport  Port=172
  vyawF2 : Outport  Port=173
  vrollF2 : Outport  Port=174
  vxF3 : Outport  Port=175
  vyF3 : Outport  Port=176
  vzF3 : Outport  Port=177
  vpitchF3 : Outport  Port=178
  vyawF3 : Outport  Port=179
  vrollF3 : Outport  Port=180
  vxBF : Outport  Port=181
  vyBF : Outport  Port=182
  vzBF : Outport  Port=183
  vpitchBF : Outport  Port=184
  vyawBF : Outport  Port=185
  vrollBF : Outport  Port=186
  vxPF : Outport  Port=187
  vyPF : Outport  Port=188
  vzPF : Outport  Port=189
  vpitchPF : Outport  Port=190
  vyawPF : Outport  Port=191
  vrollPF : Outport  Port=192
  vxMNR : Outport  Port=193
  vyMNR : Outport  Port=194
  vzMNR : Outport  Port=195
  vpitchMNR : Outport  Port=196
  vyawMNR : Outport  Port=197
  vrollMNR : Outport  Port=198
  vxMN : Outport  Port=199
  vyMN : Outport  Port=200
  vzMN : Outport  Port=201
  vpitchMN : Outport  Port=202
  vyawMN : Outport  Port=203
  vrollMN : Outport  Port=204
  vxIRM : Outport  Port=205
  vyIRM : Outport  Port=206
  vzIRM : Outport  Port=207
  vpitchIRM : Outport  Port=208
  vyawIRM : Outport  Port=209
  vrollIRM : Outport  Port=210
  vxIM : Outport  Port=211
  vyIM : Outport  Port=212
  vzIM : Outport  Port=213
  vpitchIM : Outport  Port=214
  vyawIM : Outport  Port=215
  vrollIM : Outport  Port=216
  vxRM : Outport  Port=217
  vyRM : Outport  Port=218
  vzRM : Outport  Port=219
  vpitchRM : Outport  Port=220
  vyawRM : Outport  Port=221
  vrollRM : Outport  Port=222
  vxTM : Outport  Port=223
  vyTM : Outport  Port=224
  vzTM : Outport  Port=225
  vpitchTM : Outport  Port=226
  vyawTM : Outport  Port=227
  vrollTM : Outport  Port=228
  vxHL1 : Outport  Port=229
  vyHL1 : Outport  Port=230
  vzHL1 : Outport  Port=231
  vpitchHL1 : Outport  Port=232
  vyawHL1 : Outport  Port=233
  vrollHL1 : Outport  Port=234
  vxHL2 : Outport  Port=235
  vyHL2 : Outport  Port=236
  vzHL2 : Outport  Port=237
  vpitchHL2 : Outport  Port=238
  vyawHL2 : Outport  Port=239
  vrollHL2 : Outport  Port=240
  vxHL3 : Outport  Port=241
  vyHL3 : Outport  Port=242
  vzHL3 : Outport  Port=243
  vpitchHL3 : Outport  Port=244
  vyawHL3 : Outport  Port=245
  vrollHL3 : Outport  Port=246
  vxHL21 : Outport  Port=247
  vyHL21 : Outport  Port=248
  vzHL21 : Outport  Port=249
  vpitchHL21 : Outport  Port=250
  vyawHL21 : Outport  Port=251
  vrollHL21 : Outport  Port=252
  vxHL22 : Outport  Port=253
  vyHL22 : Outport  Port=254
  vzHL22 : Outport  Port=255
  vpitchHL22 : Outport  Port=256
  vyawHL22 : Outport  Port=257
  vrollHL22 : Outport  Port=258
  vxHL23 : Outport  Port=259
  vyHL23 : Outport  Port=260
  vzHL23 : Outport  Port=261
  vpitchHL23 : Outport  Port=262
  vyawHL23 : Outport  Port=263
  vrollHL23 : Outport  Port=264
  vxJB : Outport  Port=265
  vyJB : Outport  Port=266
  vzJB : Outport  Port=267
  vpitchJB : Outport  Port=268
  vyawJB : Outport  Port=269
  vrollJB : Outport  Port=270
  wires:
  mux/1 -> SAS State-Space/1
  SAS State-Space/1 -> demux/1
  axg/1 -> mux/1
  ayg/1 -> mux/2
  azg/1 -> mux/3
  apitchg/1 -> mux/4
  ayawg/1 -> mux/5
  arollg/1 -> mux/6
  axHLgnd/1 -> mux/7
  ayHLgnd/1 -> mux/8
  azHLgnd/1 -> mux/9
  apitchHLgnd/1 -> mux/10
  ayawHLgnd/1 -> mux/11
  arollHLgnd/1 -> mux/12
  axHLgnd2/1 -> mux/13
  ayHLgnd2/1 -> mux/14
  azHLgnd2/1 -> mux/15
  apitchHLgnd2/1 -> mux/16
  ayawHLgnd2/1 -> mux/17
  arollHLgnd2/1 -> mux/18
  FxF0/1 -> mux/19
  FzF0/1 -> mux/20
  FyawF0/1 -> mux/21
  FxMD/1 -> mux/22
  FyMD/1 -> mux/23
  FzMD/1 -> mux/24
  FpitchMD/1 -> mux/25
  FyawMD/1 -> mux/26
  FrollMD/1 -> mux/27
  FxF1/1 -> mux/28
  FyF1/1 -> mux/29
  FzF1/1 -> mux/30
  FpitchF1/1 -> mux/31
  FyawF1/1 -> mux/32
  FrollF1/1 -> mux/33
  FxF2/1 -> mux/34
  FyF2/1 -> mux/35
  FzF2/1 -> mux/36
  FpitchF2/1 -> mux/37
  FyawF2/1 -> mux/38
  FrollF2/1 -> mux/39
  FxF3/1 -> mux/40
  FyF3/1 -> mux/41
  FzF3/1 -> mux/42
  FpitchF3/1 -> mux/43
  FyawF3/1 -> mux/44
  FrollF3/1 -> mux/45
  FxBF/1 -> mux/46
  FyBF/1 -> mux/47
  FzBF/1 -> mux/48
  FpitchBF/1 -> mux/49
  FyawBF/1 -> mux/50
  FrollBF/1 -> mux/51
  FxPF/1 -> mux/52
  FyPF/1 -> mux/53
  FzPF/1 -> mux/54
  FpitchPF/1 -> mux/55
  FyawPF/1 -> mux/56
  FrollPF/1 -> mux/57
  FxMNR/1 -> mux/58
  FyMNR/1 -> mux/59
  FzMNR/1 -> mux/60
  FpitchMNR/1 -> mux/61
  FyawMNR/1 -> mux/62
  FrollMNR/1 -> mux/63
  FxMN/1 -> mux/64
  FyMN/1 -> mux/65
  FzMN/1 -> mux/66
  FpitchMN/1 -> mux/67
  FyawMN/1 -> mux/68
  FrollMN/1 -> mux/69
  FxIRM/1 -> mux/70
  FyIRM/1 -> mux/71
  FzIRM/1 -> mux/72
  FpitchIRM/1 -> mux/73
  FyawIRM/1 -> mux/74
  FrollIRM/1 -> mux/75
  FxIM/1 -> mux/76
  FyIM/1 -> mux/77
  FzIM/1 -> mux/78
  FpitchIM/1 -> mux/79
  FyawIM/1 -> mux/80
  FrollIM/1 -> mux/81
  FxRM/1 -> mux/82
  FyRM/1 -> mux/83
  FzRM/1 -> mux/84
  FpitchRM/1 -> mux/85
  FyawRM/1 -> mux/86
  FrollRM/1 -> mux/87
  FxTM/1 -> mux/88
  FyTM/1 -> mux/89
  FzTM/1 -> mux/90
  FpitchTM/1 -> mux/91
  FyawTM/1 -> mux/92
  FrollTM/1 -> mux/93
  FxHL1/1 -> mux/94
  FyHL1/1 -> mux/95
  FzHL1/1 -> mux/96
  FpitchHL1/1 -> mux/97
  FyawHL1/1 -> mux/98
  FrollHL1/1 -> mux/99
  FxHL2/1 -> mux/100
  FyHL2/1 -> mux/101
  FzHL2/1 -> mux/102
  FpitchHL2/1 -> mux/103
  FyawHL2/1 -> mux/104
  FrollHL2/1 -> mux/105
  FxHL3/1 -> mux/106
  FyHL3/1 -> mux/107
  FzHL3/1 -> mux/108
  FpitchHL3/1 -> mux/109
  FyawHL3/1 -> mux/110
  FrollHL3/1 -> mux/111
  FxHL21/1 -> mux/112
  FyHL21/1 -> mux/113
  FzHL21/1 -> mux/114
  FpitchHL21/1 -> mux/115
  FyawHL21/1 -> mux/116
  FrollHL21/1 -> mux/117
  FxHL22/1 -> mux/118
  FyHL22/1 -> mux/119
  FzHL22/1 -> mux/120
  FpitchHL22/1 -> mux/121
  FyawHL22/1 -> mux/122
  FrollHL22/1 -> mux/123
  FxHL23/1 -> mux/124
  FyHL23/1 -> mux/125
  FzHL23/1 -> mux/126
  FpitchHL23/1 -> mux/127
  FyawHL23/1 -> mux/128
  FrollHL23/1 -> mux/129
  FxJB/1 -> mux/130
  FyJB/1 -> mux/131
  FzJB/1 -> mux/132
  FpitchJB/1 -> mux/133
  FyawJB/1 -> mux/134
  FrollJB/1 -> mux/135
  demux/1 -> xg/1
  demux/2 -> yg/1
  demux/3 -> zg/1
  demux/4 -> pitchg/1
  demux/5 -> yawg/1
  demux/6 -> rollg/1
  demux/7 -> xHLgnd/1
  demux/8 -> yHLgnd/1
  demux/9 -> zHLgnd/1
  demux/10 -> pitchHLgnd/1
  demux/11 -> yawHLgnd/1
  demux/12 -> rollHLgnd/1
  demux/13 -> xHLgnd2/1
  demux/14 -> yHLgnd2/1
  demux/15 -> zHLgnd2/1
  demux/16 -> pitchHLgnd2/1
  demux/17 -> yawHLgnd2/1
  demux/18 -> rollHLgnd2/1
  demux/19 -> vxg/1
  demux/20 -> vyg/1
  demux/21 -> vzg/1
  demux/22 -> vpitchg/1
  demux/23 -> vyawg/1
  demux/24 -> vrollg/1
  demux/25 -> vxHLgnd/1
  demux/26 -> vyHLgnd/1
  demux/27 -> vzHLgnd/1
  demux/28 -> vpitchHLgnd/1
  demux/29 -> vyawHLgnd/1
  demux/30 -> vrollHLgnd/1
  demux/31 -> vxHLgnd2/1
  demux/32 -> vyHLgnd2/1
  demux/33 -> vzHLgnd2/1
  demux/34 -> vpitchHLgnd2/1
  demux/35 -> vyawHLgnd2/1
  demux/36 -> vrollHLgnd2/1
  demux/37 -> xF0/1
  demux/38 -> zF0/1
  demux/39 -> yawF0/1
  demux/40 -> xMD/1
  demux/41 -> yMD/1
  demux/42 -> zMD/1
  demux/43 -> pitchMD/1
  demux/44 -> yawMD/1
  demux/45 -> rollMD/1
  demux/46 -> xF1/1
  demux/47 -> yF1/1
  demux/48 -> zF1/1
  demux/49 -> pitchF1/1
  demux/50 -> yawF1/1
  demux/51 -> rollF1/1
  demux/52 -> xF2/1
  demux/53 -> yF2/1
  demux/54 -> zF2/1
  demux/55 -> pitchF2/1
  demux/56 -> yawF2/1
  demux/57 -> rollF2/1
  demux/58 -> xF3/1
  demux/59 -> yF3/1
  demux/60 -> zF3/1
  demux/61 -> pitchF3/1
  demux/62 -> yawF3/1
  demux/63 -> rollF3/1
  demux/64 -> xBF/1
  demux/65 -> yBF/1
  demux/66 -> zBF/1
  demux/67 -> pitchBF/1
  demux/68 -> yawBF/1
  demux/69 -> rollBF/1
  demux/70 -> xPF/1
  demux/71 -> yPF/1
  demux/72 -> zPF/1
  demux/73 -> pitchPF/1
  demux/74 -> yawPF/1
  demux/75 -> rollPF/1
  demux/76 -> xMNR/1
  demux/77 -> yMNR/1
  demux/78 -> zMNR/1
  demux/79 -> pitchMNR/1
  demux/80 -> yawMNR/1
  demux/81 -> rollMNR/1
  demux/82 -> xMN/1
  demux/83 -> yMN/1
  demux/84 -> zMN/1
  demux/85 -> pitchMN/1
  demux/86 -> yawMN/1
  demux/87 -> rollMN/1
  demux/88 -> xIRM/1
  demux/89 -> yIRM/1
  demux/90 -> zIRM/1
  demux/91 -> pitchIRM/1
  demux/92 -> yawIRM/1
  demux/93 -> rollIRM/1
  demux/94 -> xIM/1
  demux/95 -> yIM/1
  demux/96 -> zIM/1
  demux/97 -> pitchIM/1
  demux/98 -> yawIM/1
  demux/99 -> rollIM/1
  demux/100 -> xRM/1
  demux/101 -> yRM/1
  demux/102 -> zRM/1
  demux/103 -> pitchRM/1
  demux/104 -> yawRM/1
  demux/105 -> rollRM/1
  demux/106 -> xTM/1
  demux/107 -> yTM/1
  demux/108 -> zTM/1
  demux/109 -> pitchTM/1
  demux/110 -> yawTM/1
  demux/111 -> rollTM/1
  demux/112 -> xHL1/1
  demux/113 -> yHL1/1
  demux/114 -> zHL1/1
  demux/115 -> pitchHL1/1
  demux/116 -> yawHL1/1
  demux/117 -> rollHL1/1
  demux/118 -> xHL2/1
  demux/119 -> yHL2/1
  demux/120 -> zHL2/1
  demux/121 -> pitchHL2/1
  demux/122 -> yawHL2/1
  demux/123 -> rollHL2/1
  demux/124 -> xHL3/1
  demux/125 -> yHL3/1
  demux/126 -> zHL3/1
  demux/127 -> pitchHL3/1
  demux/128 -> yawHL3/1
  demux/129 -> rollHL3/1
  demux/130 -> xHL21/1
  demux/131 -> yHL21/1
  demux/132 -> zHL21/1
  demux/133 -> pitchHL21/1
  demux/134 -> yawHL21/1
  demux/135 -> rollHL21/1
  demux/136 -> xHL22/1
  demux/137 -> yHL22/1
  demux/138 -> zHL22/1
  demux/139 -> pitchHL22/1
  demux/140 -> yawHL22/1
  demux/141 -> rollHL22/1
  demux/142 -> xHL23/1
  demux/143 -> yHL23/1
  demux/144 -> zHL23/1
  demux/145 -> pitchHL23/1
  demux/146 -> yawHL23/1
  demux/147 -> rollHL23/1
  demux/148 -> xJB/1
  demux/149 -> yJB/1
  demux/150 -> zJB/1
  demux/151 -> pitchJB/1
  demux/152 -> yawJB/1
  demux/153 -> rollJB/1
  demux/154 -> vxF0/1
  demux/155 -> vzF0/1
  demux/156 -> vyawF0/1
  demux/157 -> vxMD/1
  demux/158 -> vyMD/1
  demux/159 -> vzMD/1
  demux/160 -> vpitchMD/1
  demux/161 -> vyawMD/1
  demux/162 -> vrollMD/1
  demux/163 -> vxF1/1
  demux/164 -> vyF1/1
  demux/165 -> vzF1/1
  demux/166 -> vpitchF1/1
  demux/167 -> vyawF1/1
  demux/168 -> vrollF1/1
  demux/169 -> vxF2/1
  demux/170 -> vyF2/1
  demux/171 -> vzF2/1
  demux/172 -> vpitchF2/1
  demux/173 -> vyawF2/1
  demux/174 -> vrollF2/1
  demux/175 -> vxF3/1
  demux/176 -> vyF3/1
  demux/177 -> vzF3/1
  demux/178 -> vpitchF3/1
  demux/179 -> vyawF3/1
  demux/180 -> vrollF3/1
  demux/181 -> vxBF/1
  demux/182 -> vyBF/1
  demux/183 -> vzBF/1
  demux/184 -> vpitchBF/1
  demux/185 -> vyawBF/1
  demux/186 -> vrollBF/1
  demux/187 -> vxPF/1
  demux/188 -> vyPF/1
  demux/189 -> vzPF/1
  demux/190 -> vpitchPF/1
  demux/191 -> vyawPF/1
  demux/192 -> vrollPF/1
  demux/193 -> vxMNR/1
  demux/194 -> vyMNR/1
  demux/195 -> vzMNR/1
  demux/196 -> vpitchMNR/1
  demux/197 -> vyawMNR/1
  demux/198 -> vrollMNR/1
  demux/199 -> vxMN/1
  demux/200 -> vyMN/1
  demux/201 -> vzMN/1
  demux/202 -> vpitchMN/1
  demux/203 -> vyawMN/1
  demux/204 -> vrollMN/1
  demux/205 -> vxIRM/1
  demux/206 -> vyIRM/1
  demux/207 -> vzIRM/1
  demux/208 -> vpitchIRM/1
  demux/209 -> vyawIRM/1
  demux/210 -> vrollIRM/1
  demux/211 -> vxIM/1
  demux/212 -> vyIM/1
  demux/213 -> vzIM/1
  demux/214 -> vpitchIM/1
  demux/215 -> vyawIM/1
  demux/216 -> vrollIM/1
  demux/217 -> vxRM/1
  demux/218 -> vyRM/1
  demux/219 -> vzRM/1
  demux/220 -> vpitchRM/1
  demux/221 -> vyawRM/1
  demux/222 -> vrollRM/1
  demux/223 -> vxTM/1
  demux/224 -> vyTM/1
  demux/225 -> vzTM/1
  demux/226 -> vpitchTM/1
  demux/227 -> vyawTM/1
  demux/228 -> vrollTM/1
  demux/229 -> vxHL1/1
  demux/230 -> vyHL1/1
  demux/231 -> vzHL1/1
  demux/232 -> vpitchHL1/1
  demux/233 -> vyawHL1/1
  demux/234 -> vrollHL1/1
  demux/235 -> vxHL2/1
  demux/236 -> vyHL2/1
  demux/237 -> vzHL2/1
  demux/238 -> vpitchHL2/1
  demux/239 -> vyawHL2/1
  demux/240 -> vrollHL2/1
  demux/241 -> vxHL3/1
  demux/242 -> vyHL3/1
  demux/243 -> vzHL3/1
  demux/244 -> vpitchHL3/1
  demux/245 -> vyawHL3/1
  demux/246 -> vrollHL3/1
  demux/247 -> vxHL21/1
  demux/248 -> vyHL21/1
  demux/249 -> vzHL21/1
  demux/250 -> vpitchHL21/1
  demux/251 -> vyawHL21/1
  demux/252 -> vrollHL21/1
  demux/253 -> vxHL22/1
  demux/254 -> vyHL22/1
  demux/255 -> vzHL22/1
  demux/256 -> vpitchHL22/1
  demux/257 -> vyawHL22/1
  demux/258 -> vrollHL22/1
  demux/259 -> vxHL23/1
  demux/260 -> vyHL23/1
  demux/261 -> vzHL23/1
  demux/262 -> vpitchHL23/1
  demux/263 -> vyawHL23/1
  demux/264 -> vrollHL23/1
  demux/265 -> vxJB/1
  demux/266 -> vyJB/1
  demux/267 -> vzJB/1
  demux/268 -> vpitchJB/1
  demux/269 -> vyawJB/1
  demux/270 -> vrollJB/1
